simulink model "C172S_IntegratedAutopilot_V1"  (R2026a)
settings: Solver=ode4  StartTime=0  StopTime=180  FixedStep=0.01
InitFcn:
  | ah1Data = c172sLongitudinalData();
  | [~,ah1Plant] = c172sLongitudinalPlant(ah1Data);
  | ah1PitchController = c172sPitchAttitudeControllerData();
  | ah1Actuator = c172sElevatorActuatorData();
  | ah1AltitudeController = c172sAltitudeHoldControllerData();
  | A_ah1 = ah1Plant.A; B_ah1 = ah1Plant.B;
  | C_ah1 = ah1Plant.C; D_ah1 = ah1Plant.D;
  | Vtrim_ah1_mps = ah1Data.trim.V_mps;
  | Kh_ah1_per_s = ah1AltitudeController.altitudeGain_per_s;
  | Kv_ah1_radPerMps = ah1AltitudeController.verticalSpeedGain_radPerMps;
  | tauAltitude_ah1_s = ah1AltitudeController.commandFilterTimeConstant_s;
  | hDotLimit_ah1_mps = ah1AltitudeController.verticalSpeedCommandLimit_mps;
  | thetaLimit_ah1_rad = ah1AltitudeController.pitchCommandLimit_rad;
  | Kp_ah1 = ah1PitchController.Kp_radPerRad;
  | Ki_ah1_per_s = ah1PitchController.Ki_radPerRadPerS;
  | Kq_ah1_s = ah1Actuator.integration.Kq_s;
  | tauTheta_ah1_s = ah1PitchController.commandFilterTimeConstant_s;
  | tauActuator_ah1_s = ah1Actuator.dynamics.timeConstant_s;
  | Tt_ah1_s = ah1Actuator.antiWindup.trackingTimeConstant_s;
  | deltaELower_ah1_rad = ah1Actuator.authority.lowerLimit_rad;
  | deltaEUpper_ah1_rad = ah1Actuator.authority.upperLimit_rad;
  | deltaERate_ah1_radps = deg2rad(ah1Actuator.dynamics.rateLimit_degps);
  | if ~exist('hCommand_ah1_m','var'), hCommand_ah1_m = ah1AltitudeController.validation.operationalCommand_m; end
  | if ~exist('antiWindupEnable_ah1','var'), antiWindupEnable_ah1 = 1.0; end
  | if ~exist('x0_ah1','var'), x0_ah1 = zeros(4,1); end
  | if ~exist('xi0_ah1','var'), xi0_ah1 = 0.0; end
  | if ~exist('deltaE0_ah1','var'), deltaE0_ah1 = 0.0; end
  | if ~exist('h0_ah1_m','var'), h0_ah1_m = 0.0; end
  | hh1Data = c172sLateralDirectionalData();
  | [~,hh1Plant] = c172sLateralDirectionalPlant(hh1Data);
  | hh1YawController = c172sYawDamperData();
  | hh1RudderActuator = c172sRudderActuatorData();
  | hh1RollController = c172sRollAttitudeControllerData();
  | hh1AileronActuator = c172sAileronActuatorData();
  | hh1HeadingSensor = c172sHeadingSensorData();
  | hh1HeadingController = c172sHeadingHoldControllerData();
  | if ~strcmp(hh1Data.model.version,hh1HeadingController.requiredPlantVersion), error('HH V1 plant dependency mismatch.'); end
  | if ~strcmp(hh1YawController.artifactRevision,hh1HeadingController.requiredYawDamperRevision), error('HH V1 yaw-controller dependency mismatch.'); end
  | if ~strcmp(hh1RudderActuator.artifactRevision,hh1HeadingController.requiredRudderAuditRevision), error('HH V1 rudder-audit dependency mismatch.'); end
  | if ~strcmp(hh1AileronActuator.artifactRevision,hh1HeadingController.requiredAileronAuditRevision), error('HH V1 aileron-audit dependency mismatch.'); end
  | if ~strcmp(hh1RollController.artifactRevision,hh1HeadingController.requiredRollControllerRevision), error('HH V1 roll-controller dependency mismatch.'); end
  | if ~strcmp(hh1HeadingSensor.artifactRevision,hh1HeadingController.requiredHeadingSensorRevision), error('HH V1 heading-sensor dependency mismatch.'); end
  | A_hh1 = hh1Plant.A; B_hh1 = hh1Plant.B;
  | C_hh1 = hh1Plant.C; D_hh1 = hh1Plant.D;
  | Kphi_hh1 = hh1RollController.bankProportionalGain;
  | Ki_hh1 = hh1RollController.bankIntegralGain_per_s;
  | Kp_hh1 = hh1RollController.rollRateGain_s;
  | Tcmd_hh1 = hh1RollController.commandFilterTimeConstant_s;
  | Kr_hh1 = hh1YawController.rudderGain_s;
  | Tw_hh1 = hh1YawController.washoutTimeConstant_s;
  | TsRudder_hh1 = hh1RudderActuator.sensor.filterTimeConstant_s;
  | tauRudder_hh1 = hh1RudderActuator.dynamics.timeConstant_s;
  | TsRoll_hh1 = hh1AileronActuator.sensor.filterTimeConstant_s;
  | tauAileron_hh1 = hh1AileronActuator.dynamics.timeConstant_s;
  | Tt_hh1 = hh1AileronActuator.antiWindup.trackingTimeConstant_s;
  | delaySampleTime_hh1 = hh1AileronActuator.sensor.nominalDelay_s;
  | Kpsi_hh1 = hh1HeadingController.headingErrorGain;
  | TsHeading_hh1 = hh1HeadingSensor.filterTimeConstant_s;
  | headingDelaySampleTime_hh1 = hh1HeadingSensor.nominalDelay_s/5;
  | bankCommandLower_hh1_rad = -deg2rad(hh1HeadingController.bankCommandAuthority_deg);
  | bankCommandUpper_hh1_rad = deg2rad(hh1HeadingController.bankCommandAuthority_deg);
  | autoAileronLower_hh1_rad = hh1AileronActuator.authority.lowerLimit_rad;
  | autoAileronUpper_hh1_rad = hh1AileronActuator.authority.upperLimit_rad;
  | aileronRateLower_hh1_radps = -deg2rad(hh1AileronActuator.dynamics.rateLimit_degps);
  | aileronRateUpper_hh1_radps = deg2rad(hh1AileronActuator.dynamics.rateLimit_degps);
  | totalAileronLower_hh1_rad = hh1AileronActuator.physicalTravel.lowerLimit_rad;
  | totalAileronUpper_hh1_rad = hh1AileronActuator.physicalTravel.upperLimit_rad;
  | autoRudderLower_hh1_rad = hh1RudderActuator.authority.lowerLimit_rad;
  | autoRudderUpper_hh1_rad = hh1RudderActuator.authority.upperLimit_rad;
  | rudderRateLower_hh1_radps = -deg2rad(hh1RudderActuator.dynamics.rateLimit_degps);
  | rudderRateUpper_hh1_radps = deg2rad(hh1RudderActuator.dynamics.rateLimit_degps);
  | totalRudderLower_hh1_rad = hh1RudderActuator.physicalTravel.lowerLimit_rad;
  | totalRudderUpper_hh1_rad = hh1RudderActuator.physicalTravel.upperLimit_rad;
  | if ~exist('headingCommand_hh1_rad','var'), headingCommand_hh1_rad = deg2rad(30); end
  | if ~exist('headingBias_hh1_rad','var'), headingBias_hh1_rad = 0; end
  | if ~exist('headingNoiseAmplitude_hh1_rad','var'), headingNoiseAmplitude_hh1_rad = 0; end
  | if ~exist('headingNoiseFrequency_hh1_radps','var'), headingNoiseFrequency_hh1_radps = 0.8; end
  | if ~exist('pilotAileronBias_hh1_rad','var'), pilotAileronBias_hh1_rad = 0; end
  | if ~exist('pilotAileronPulse_hh1_rad','var'), pilotAileronPulse_hh1_rad = 0; end
  | if ~exist('pilotRudderBias_hh1_rad','var'), pilotRudderBias_hh1_rad = 0; end
  | if ~exist('pilotRudderPulse_hh1_rad','var'), pilotRudderPulse_hh1_rad = 0; end
  | if ~exist('aileronPulseStart_hh1_s','var'), aileronPulseStart_hh1_s = 5; end
  | if ~exist('aileronPulseEnd_hh1_s','var'), aileronPulseEnd_hh1_s = 6; end
  | if ~exist('rudderPulseStart_hh1_s','var'), rudderPulseStart_hh1_s = 5; end
  | if ~exist('rudderPulseEnd_hh1_s','var'), rudderPulseEnd_hh1_s = 6; end
  | if ~exist('pNoiseAmplitude_hh1_radps','var'), pNoiseAmplitude_hh1_radps = 0; end
  | if ~exist('pNoiseFrequency_hh1_radps','var'), pNoiseFrequency_hh1_radps = 50; end
  | if ~exist('phiNoiseAmplitude_hh1_rad','var'), phiNoiseAmplitude_hh1_rad = 0; end
  | if ~exist('phiNoiseFrequency_hh1_radps','var'), phiNoiseFrequency_hh1_radps = 5; end
  | if ~exist('yawNoiseAmplitude_hh1_radps','var'), yawNoiseAmplitude_hh1_radps = 0; end
  | if ~exist('yawNoiseFrequency_hh1_radps','var'), yawNoiseFrequency_hh1_radps = 50; end
  | if ~exist('antiWindupEnable_hh1','var'), antiWindupEnable_hh1 = 1; end
  | if ~exist('x0_hh1','var'), x0_hh1 = zeros(5,1); end
  | if ~exist('rDelay0_hh1_radps','var'), rDelay0_hh1_radps = x0_hh1(3); end
  | if ~exist('pDelay0_hh1_radps','var'), pDelay0_hh1_radps = x0_hh1(2); end
  | if ~exist('phiDelay0_hh1_rad','var'), phiDelay0_hh1_rad = x0_hh1(4); end
  | if ~exist('rSensor0_hh1_radps','var'), rSensor0_hh1_radps = 0; end
  | if ~exist('xw0_hh1_radps','var'), xw0_hh1_radps = 0; end
  | if ~exist('deltaRAuto0_hh1_rad','var'), deltaRAuto0_hh1_rad = 0; end
  | if ~exist('pSensor0_hh1_radps','var'), pSensor0_hh1_radps = 0; end
  | if ~exist('phiSensor0_hh1_rad','var'), phiSensor0_hh1_rad = 0; end
  | if ~exist('psiDelay0_hh1_rad','var'), psiDelay0_hh1_rad = x0_hh1(5); end
  | if ~exist('psiSensor0_hh1_rad','var'), psiSensor0_hh1_rad = x0_hh1(5)+headingBias_hh1_rad; end
  | if ~exist('xi0_hh1_rad_s','var'), xi0_hh1_rad_s = 0; end
  | if ~exist('deltaAAuto0_hh1_rad','var'), deltaAAuto0_hh1_rad = 0; end
  | if ~exist('filteredCommand0_hh1_rad','var'), filteredCommand0_hh1_rad = 0; end
  | ia1Integration = c172sIntegratedAutopilotData();
  | if ~strcmp(ia1Integration.artifactRevision,'INTEGRATED-AUTOPILOT-V1-INTERFACE-AUDIT-MATLAB-R1'), error('Integrated Autopilot V1 audit mismatch.'); end
  | if ~exist('ia1InputSignal','var'), error('ia1InputSignal is required.'); end
  | ia1TrimAltitude_ft = 4000.0;
undefined symbols (not defined in the file or in its folder): aileronPulseEnd_hh1_s, aileronPulseStart_hh1_s, antiWindupEnable_ah1, antiWindupEnable_hh1, deltaAAuto0_hh1_rad, deltaE0_ah1, deltaRAuto0_hh1_rad, filteredCommand0_hh1_rad, h0_ah1_m, headingBias_hh1_rad, headingNoiseAmplitude_hh1_rad, headingNoiseFrequency_hh1_radps, pDelay0_hh1_radps, phiDelay0_hh1_rad, phiNoiseAmplitude_hh1_rad, phiNoiseFrequency_hh1_radps, phiSensor0_hh1_rad, pilotAileronBias_hh1_rad, pilotAileronPulse_hh1_rad, pilotRudderBias_hh1_rad, pilotRudderPulse_hh1_rad, pNoiseAmplitude_hh1_radps, pNoiseFrequency_hh1_radps, pSensor0_hh1_radps, psiDelay0_hh1_rad, psiSensor0_hh1_rad, rDelay0_hh1_radps, rSensor0_hh1_radps, rudderPulseEnd_hh1_s, rudderPulseStart_hh1_s, x0_ah1, x0_hh1, xi0_ah1, xi0_hh1_rad_s, xw0_hh1_radps, yawNoiseAmplitude_hh1_radps, yawNoiseFrequency_hh1_radps
(part 1 of 2)
settings Model: Creator=Shahi  LastModifiedBy=Shahi

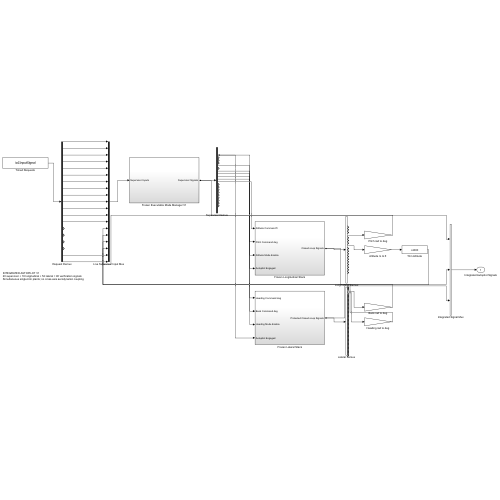
[thumbnail: Simulink's stored preview of the top-level diagram]
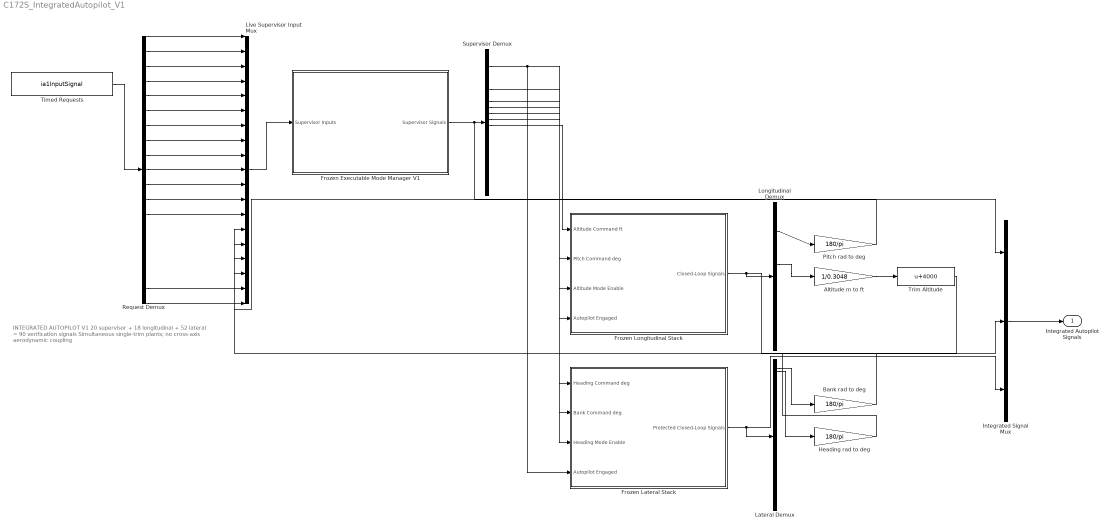
== system C172S_IntegratedAutopilot_V1 ==
  note: INTEGRATED AUTOPILOT V1
      | 20 supervisor + 18 longitudinal + 52 lateral = 90 verification signals
      | Simultaneous single-trim plants; no cross-axis aerodynamic coupling
  Altitude m to ft : Gain  Gain=1/0.3048
  Bank rad to deg : Gain  Gain=180/pi
  Frozen Executable Mode Manager V1 : Subsystem
  Frozen Lateral Stack : Subsystem
  Frozen Longitudinal Stack : Subsystem
  Heading rad to deg : Gain  Gain=180/pi
  Integrated Signal Mux : Mux  Inputs=3
  Lateral Demux : Demux  Outputs=52
  Live Supervisor Input Mux : Mux  Inputs=19
  Longitudinal Demux : Demux  Outputs=18
  Pitch rad to deg : Gain  Gain=180/pi
  Request Demux : Demux  Outputs=19
  Supervisor Demux : Demux  Outputs=20
  Timed Requests : FromWorkspace  VariableName=ia1InputSignal  SampleTime=0.01  Interpolate=off  OutputAfterFinalValue=Holding final value
  Trim Altitude : Bias  Bias=4000  SaturateOnIntegerOverflow=off
  Integrated Autopilot Signals : Outport
  wires:
  Timed Requests/1 -> Request Demux/1
  Frozen Longitudinal Stack/1(Closed-Loop Signals) -> Longitudinal Demux/1, Integrated Signal Mux/2
  Frozen Lateral Stack/1(Protected Closed-Loop Signals) -> Lateral Demux/1, Integrated Signal Mux/3
  Longitudinal Demux/4 -> Pitch rad to deg/1
  Longitudinal Demux/8 -> Altitude m to ft/1
  Altitude m to ft/1 -> Trim Altitude/1
  Lateral Demux/4 -> Bank rad to deg/1
  Lateral Demux/5 -> Heading rad to deg/1
  Request Demux/1 -> Live Supervisor Input Mux/1
  Request Demux/2 -> Live Supervisor Input Mux/2
  Request Demux/3 -> Live Supervisor Input Mux/3
  Request Demux/4 -> Live Supervisor Input Mux/4
  Request Demux/5 -> Live Supervisor Input Mux/5
  Request Demux/6 -> Live Supervisor Input Mux/6
  Request Demux/7 -> Live Supervisor Input Mux/7
  Request Demux/8 -> Live Supervisor Input Mux/8
  Request Demux/9 -> Live Supervisor Input Mux/9
  Request Demux/10 -> Live Supervisor Input Mux/10
  Request Demux/11 -> Live Supervisor Input Mux/11
  Request Demux/12 -> Live Supervisor Input Mux/12
  Request Demux/13 -> Live Supervisor Input Mux/13
  Request Demux/18 -> Live Supervisor Input Mux/18
  Request Demux/19 -> Live Supervisor Input Mux/19
  Bank rad to deg/1 -> Live Supervisor Input Mux/14
  Pitch rad to deg/1 -> Live Supervisor Input Mux/15
  Heading rad to deg/1 -> Live Supervisor Input Mux/16
  Trim Altitude/1 -> Live Supervisor Input Mux/17
  Live Supervisor Input Mux/1 -> Frozen Executable Mode Manager V1/1(Supervisor Inputs)
  Frozen Executable Mode Manager V1/1(Supervisor Signals) -> Supervisor Demux/1, Integrated Signal Mux/1
  Supervisor Demux/11 -> Frozen Longitudinal Stack/1(Altitude Command ft)
  Supervisor Demux/9 -> Frozen Longitudinal Stack/2(Pitch Command deg)
  Supervisor Demux/7 -> Frozen Longitudinal Stack/3(Altitude Mode Enable)
  Supervisor Demux/1 -> Frozen Longitudinal Stack/4(Autopilot Engaged), Frozen Lateral Stack/4(Autopilot Engaged)
  Supervisor Demux/10 -> Frozen Lateral Stack/1(Heading Command deg)
  Supervisor Demux/8 -> Frozen Lateral Stack/2(Bank Command deg)
  Supervisor Demux/5 -> Frozen Lateral Stack/3(Heading Mode Enable)
  Integrated Signal Mux/1 -> Integrated Autopilot Signals/1

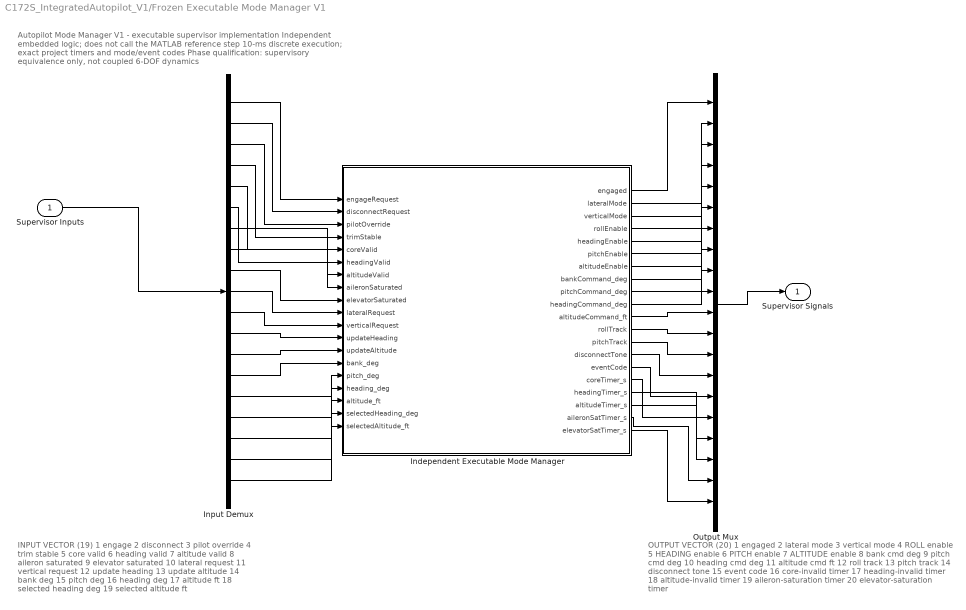
== system C172S_IntegratedAutopilot_V1/Frozen Executable Mode Manager V1 ==
  note: Autopilot Mode Manager V1 - executable supervisor implementation
      | Independent embedded logic; does not call the MATLAB reference step
      | 10-ms discrete execution; exact project timers and mode/event codes
      | Phase qualification: supervisory equivalence only, not coupled 6-DOF dynamics
  note: INPUT VECTOR (19)
      | 1 engage  2 disconnect  3 pilot override  4 trim stable
      | 5 core valid  6 heading valid  7 altitude valid
      | 8 aileron saturated  9 elevator saturated
      | 10 lateral request  11 vertical request
      | 12 update heading  13 update altitude
      | 14 bank deg  15 pitch deg  16 heading deg  17 altitude ft
      | 18 selected heading deg  19 selected altitude ft
  note: OUTPUT VECTOR (20)
      | 1 engaged  2 lateral mode  3 vertical mode
      | 4 ROLL enable  5 HEADING enable  6 PITCH enable  7 ALTITUDE enable
      | 8 bank cmd deg  9 pitch cmd deg  10 heading cmd deg  11 altitude cmd ft
      | 12 roll track  13 pitch track  14 disconnect tone  15 event code
      | 16 core-invalid timer  17 heading-invalid timer  18 altitude-invalid timer
      | 19 aileron-saturation timer  20 elevator-saturation timer
  Supervisor Inputs : Inport
  Independent Executable Mode Manager : MATLAB Function  TreatAsAtomicUnit=on
  Input Demux : Demux  Outputs=19
  Output Mux : Mux  Inputs=20
  Supervisor Signals : Outport
  wires:
  Input Demux/1 -> Independent Executable Mode Manager/1(engageRequest)
  Input Demux/2 -> Independent Executable Mode Manager/2(disconnectRequest)
  Input Demux/3 -> Independent Executable Mode Manager/3(pilotOverride)
  Input Demux/4 -> Independent Executable Mode Manager/4(trimStable)
  Input Demux/5 -> Independent Executable Mode Manager/5(coreValid)
  Input Demux/6 -> Independent Executable Mode Manager/6(headingValid)
  Input Demux/7 -> Independent Executable Mode Manager/7(altitudeValid)
  Input Demux/8 -> Independent Executable Mode Manager/8(aileronSaturated)
  Input Demux/9 -> Independent Executable Mode Manager/9(elevatorSaturated)
  Input Demux/10 -> Independent Executable Mode Manager/10(lateralRequest)
  Input Demux/11 -> Independent Executable Mode Manager/11(verticalRequest)
  Input Demux/12 -> Independent Executable Mode Manager/12(updateHeading)
  Input Demux/13 -> Independent Executable Mode Manager/13(updateAltitude)
  Input Demux/14 -> Independent Executable Mode Manager/14(bank_deg)
  Input Demux/15 -> Independent Executable Mode Manager/15(pitch_deg)
  Input Demux/16 -> Independent Executable Mode Manager/16(heading_deg)
  Input Demux/17 -> Independent Executable Mode Manager/17(altitude_ft)
  Input Demux/18 -> Independent Executable Mode Manager/18(selectedHeading_deg)
  Input Demux/19 -> Independent Executable Mode Manager/19(selectedAltitude_ft)
  Independent Executable Mode Manager/1(engaged) -> Output Mux/1
  Independent Executable Mode Manager/2(lateralMode) -> Output Mux/2
  Independent Executable Mode Manager/3(verticalMode) -> Output Mux/3
  Independent Executable Mode Manager/4(rollEnable) -> Output Mux/4
  Independent Executable Mode Manager/5(headingEnable) -> Output Mux/5
  Independent Executable Mode Manager/6(pitchEnable) -> Output Mux/6
  Independent Executable Mode Manager/7(altitudeEnable) -> Output Mux/7
  Independent Executable Mode Manager/8(bankCommand_deg) -> Output Mux/8
  Independent Executable Mode Manager/9(pitchCommand_deg) -> Output Mux/9
  Independent Executable Mode Manager/10(headingCommand_deg) -> Output Mux/10
  Independent Executable Mode Manager/11(altitudeCommand_ft) -> Output Mux/11
  Independent Executable Mode Manager/12(rollTrack) -> Output Mux/12
  Independent Executable Mode Manager/13(pitchTrack) -> Output Mux/13
  Independent Executable Mode Manager/14(disconnectTone) -> Output Mux/14
  Independent Executable Mode Manager/15(eventCode) -> Output Mux/15
  Independent Executable Mode Manager/16(coreTimer_s) -> Output Mux/16
  Independent Executable Mode Manager/17(headingTimer_s) -> Output Mux/17
  Independent Executable Mode Manager/18(altitudeTimer_s) -> Output Mux/18
  Independent Executable Mode Manager/19(aileronSatTimer_s) -> Output Mux/19
  Independent Executable Mode Manager/20(elevatorSatTimer_s) -> Output Mux/20
  Output Mux/1 -> Supervisor Signals/1
  Supervisor Inputs/1 -> Input Demux/1

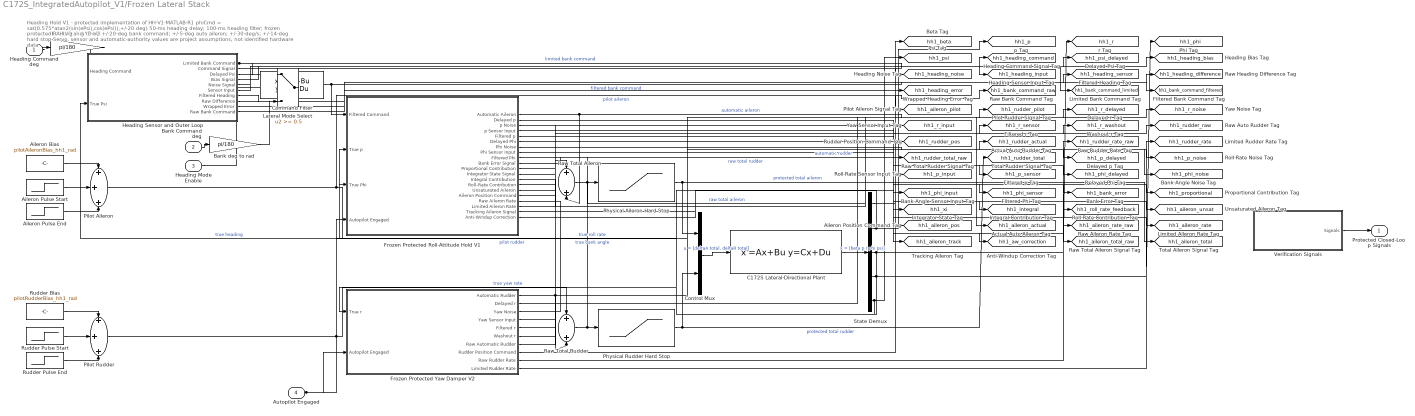
== system C172S_IntegratedAutopilot_V1/Frozen Lateral Stack ==
  note: Heading Hold V1 - protected implementation of HH-V1-MATLAB-R1
      | phiCmd = sat(0.575*atan2(sin(ePsi),cos(ePsi)),+/-20 deg)
      | 50-ms heading delay; 100-ms heading filter; frozen protected RAH V1 and YD V2
      | +/-20-deg bank command; +/-5-deg auto aileron; +/-30-deg/s; +/-14-deg hard stop
      | Servo, sensor and automatic-authority values are project assumptions, not identified hardware data
  Heading Command deg : Inport
  Bank Command deg : Inport  Port=2
  Heading Mode Enable : Inport  Port=3
  Autopilot Engaged : Inport  Port=4
  Aileron Bias : Constant  Value=pilotAileronBias_hh1_rad
  Aileron Pulse End : Step  Time=aileronPulseEnd_hh1_s  FinalValue=-pilotAileronPulse_hh1_rad  SampleTime=0
  Aileron Pulse Start : Step  Time=aileronPulseStart_hh1_s  FinalValue=pilotAileronPulse_hh1_rad  SampleTime=0
  Bank deg to rad : Gain  Gain=pi/180
  C172S Lateral-Directional Plant : StateSpace  A=A_hh1  B=B_hh1  C=C_hh1  D=D_hh1  InitialCondition=x0_hh1
  Command Filter : StateSpace  A=-1/Tcmd_hh1  B=1/Tcmd_hh1  D=0  InitialCondition=filteredCommand0_hh1_rad
  Control Mux : Mux  Inputs=2
  Frozen Protected Roll-Attitude Hold V1 : Subsystem
  Frozen Protected Yaw Damper V2 : Subsystem
  Heading Sensor and Outer Loop : Subsystem
  Heading deg to rad : Gain  Gain=pi/180
  Lateral Mode Select : Switch  Threshold=0.5  SaturateOnIntegerOverflow=off  InputSameDT=off
  Physical Aileron Hard Stop : Saturate  UpperLimit=totalAileronUpper_hh1_rad  LowerLimit=totalAileronLower_hh1_rad
  Physical Rudder Hard Stop : Saturate  UpperLimit=totalRudderUpper_hh1_rad  LowerLimit=totalRudderLower_hh1_rad
  Pilot Aileron : Sum  Inputs=+++
  Pilot Rudder : Sum  Inputs=+++
  Raw Total Aileron : Sum
  Raw Total Rudder : Sum
  Rudder Bias : Constant  Value=pilotRudderBias_hh1_rad
  Rudder Pulse End : Step  Time=rudderPulseEnd_hh1_s  FinalValue=-pilotRudderPulse_hh1_rad  SampleTime=0
  Rudder Pulse Start : Step  Time=rudderPulseStart_hh1_s  FinalValue=pilotRudderPulse_hh1_rad  SampleTime=0
  State Demux : Demux  Outputs=5
  Verification Signals : Subsystem
  Protected Closed-Loop Signals : Outport
  tag scope: hh1_aileron_actual=global, hh1_aileron_pilot=global, hh1_aileron_pos=global, hh1_aileron_rate=global, hh1_aileron_rate_raw=global, hh1_aileron_total=global, hh1_aileron_total_raw=global, hh1_aileron_track=global, hh1_aileron_unsat=global, hh1_aw_correction=global, hh1_bank_command_filtered=global, hh1_bank_command_limited=global, hh1_bank_command_raw=global, hh1_bank_error=global, hh1_beta=global, hh1_heading_bias=global, hh1_heading_command=global, hh1_heading_difference=global, hh1_heading_error=global, hh1_heading_input=global, hh1_heading_noise=global, hh1_heading_sensor=global, hh1_integral=global, hh1_p=global, hh1_p_delayed=global, hh1_p_input=global, hh1_p_noise=global, hh1_p_sensor=global, hh1_phi=global, hh1_phi_delayed=global, hh1_phi_input=global, hh1_phi_noise=global, hh1_phi_sensor=global, hh1_proportional=global, hh1_psi=global, hh1_psi_delayed=global, hh1_r=global, hh1_r_delayed=global, hh1_r_input=global, hh1_r_noise=global, hh1_r_sensor=global, hh1_r_washout=global, hh1_roll_rate_feedback=global, hh1_rudder_actual=global, hh1_rudder_pilot=global, hh1_rudder_pos=global, hh1_rudder_rate=global, hh1_rudder_rate_raw=global, hh1_rudder_raw=global, hh1_rudder_total=global, hh1_rudder_total_raw=global, hh1_xi=global
  wires:
  Heading Sensor and Outer Loop/1(Limited Bank Command) -> [hh1_bank_command_limited], Lateral Mode Select/1  "limited bank command"
  Command Filter/1 -> [hh1_bank_command_filtered], Frozen Protected Roll-Attitude Hold V1/1(Filtered Command)  "filtered bank command"
  Aileron Bias/1 -> Pilot Aileron/1
  Aileron Pulse Start/1 -> Pilot Aileron/2
  Aileron Pulse End/1 -> Pilot Aileron/3
  Rudder Bias/1 -> Pilot Rudder/1
  Rudder Pulse Start/1 -> Pilot Rudder/2
  Rudder Pulse End/1 -> Pilot Rudder/3
  Pilot Aileron/1 -> [hh1_aileron_pilot], Raw Total Aileron/1  "pilot aileron"
  Frozen Protected Roll-Attitude Hold V1/1(Automatic Aileron) -> [hh1_aileron_actual], Raw Total Aileron/2  "automatic aileron"
  Raw Total Aileron/1 -> [hh1_aileron_total_raw], Physical Aileron Hard Stop/1  "raw total aileron"
  Physical Aileron Hard Stop/1 -> [hh1_aileron_total], Control Mux/1  "protected total aileron"
  Pilot Rudder/1 -> [hh1_rudder_pilot], Raw Total Rudder/1  "pilot rudder"
  Frozen Protected Yaw Damper V2/1(Automatic Rudder) -> [hh1_rudder_actual], Raw Total Rudder/2  "automatic rudder"
  Raw Total Rudder/1 -> [hh1_rudder_total_raw], Physical Rudder Hard Stop/1  "raw total rudder"
  Physical Rudder Hard Stop/1 -> [hh1_rudder_total], Control Mux/2  "protected total rudder"
  Control Mux/1 -> C172S Lateral-Directional Plant/1  "u = [deltaA total, deltaR total]"
  C172S Lateral-Directional Plant/1 -> State Demux/1  "x = [beta p r phi psi]"
  State Demux/2 -> [hh1_p], Frozen Protected Roll-Attitude Hold V1/2(True p)  "true roll rate"
  State Demux/4 -> [hh1_phi], Frozen Protected Roll-Attitude Hold V1/3(True Phi)  "true bank angle"
  State Demux/3 -> [hh1_r], Frozen Protected Yaw Damper V2/1(True r)  "true yaw rate"
  State Demux/5 -> [hh1_psi], Heading Sensor and Outer Loop/2(True Psi)  "true heading"
  Verification Signals/1(Signals) -> Protected Closed-Loop Signals/1
  State Demux/1 -> [hh1_beta]
  Heading Sensor and Outer Loop/2(Command Signal) -> [hh1_heading_command]
  Heading Sensor and Outer Loop/3(Delayed Psi) -> [hh1_psi_delayed]
  Heading Sensor and Outer Loop/4(Bias Signal) -> [hh1_heading_bias]
  Heading Sensor and Outer Loop/5(Noise Signal) -> [hh1_heading_noise]
  Heading Sensor and Outer Loop/6(Sensor Input) -> [hh1_heading_input]
  Heading Sensor and Outer Loop/7(Filtered Heading) -> [hh1_heading_sensor]
  Heading Sensor and Outer Loop/8(Raw Difference) -> [hh1_heading_difference]
  Heading Sensor and Outer Loop/9(Wrapped Error) -> [hh1_heading_error]
  Heading Sensor and Outer Loop/10(Raw Bank Command) -> [hh1_bank_command_raw]
  Frozen Protected Yaw Damper V2/2(Delayed r) -> [hh1_r_delayed]
  Frozen Protected Yaw Damper V2/3(Yaw Noise) -> [hh1_r_noise]
  Frozen Protected Yaw Damper V2/4(Yaw Sensor Input) -> [hh1_r_input]
  Frozen Protected Yaw Damper V2/5(Filtered r) -> [hh1_r_sensor]
  Frozen Protected Yaw Damper V2/6(Washout r) -> [hh1_r_washout]
  Frozen Protected Yaw Damper V2/7(Raw Automatic Rudder) -> [hh1_rudder_raw]
  Frozen Protected Yaw Damper V2/8(Rudder Position Command) -> [hh1_rudder_pos]
  Frozen Protected Yaw Damper V2/9(Raw Rudder Rate) -> [hh1_rudder_rate_raw]
  Frozen Protected Yaw Damper V2/10(Limited Rudder Rate) -> [hh1_rudder_rate]
  Frozen Protected Roll-Attitude Hold V1/2(Delayed p) -> [hh1_p_delayed]
  Frozen Protected Roll-Attitude Hold V1/3(p Noise) -> [hh1_p_noise]
  Frozen Protected Roll-Attitude Hold V1/4(p Sensor Input) -> [hh1_p_input]
  Frozen Protected Roll-Attitude Hold V1/5(Filtered p) -> [hh1_p_sensor]
  Frozen Protected Roll-Attitude Hold V1/6(Delayed Phi) -> [hh1_phi_delayed]
  Frozen Protected Roll-Attitude Hold V1/7(Phi Noise) -> [hh1_phi_noise]
  Frozen Protected Roll-Attitude Hold V1/8(Phi Sensor Input) -> [hh1_phi_input]
  Frozen Protected Roll-Attitude Hold V1/9(Filtered Phi) -> [hh1_phi_sensor]
  Frozen Protected Roll-Attitude Hold V1/10(Bank Error Signal) -> [hh1_bank_error]
  Frozen Protected Roll-Attitude Hold V1/11(Proportional Contribution) -> [hh1_proportional]
  Frozen Protected Roll-Attitude Hold V1/12(Integrator State Signal) -> [hh1_xi]
  Frozen Protected Roll-Attitude Hold V1/13(Integral Contribution) -> [hh1_integral]
  Frozen Protected Roll-Attitude Hold V1/14(Roll-Rate Contribution) -> [hh1_roll_rate_feedback]
  Frozen Protected Roll-Attitude Hold V1/15(Unsaturated Aileron) -> [hh1_aileron_unsat]
  Frozen Protected Roll-Attitude Hold V1/16(Aileron Position Command) -> [hh1_aileron_pos]
  Frozen Protected Roll-Attitude Hold V1/17(Raw Aileron Rate) -> [hh1_aileron_rate_raw]
  Frozen Protected Roll-Attitude Hold V1/18(Limited Aileron Rate) -> [hh1_aileron_rate]
  Frozen Protected Roll-Attitude Hold V1/19(Tracking Aileron Signal) -> [hh1_aileron_track]
  Frozen Protected Roll-Attitude Hold V1/20(Anti-Windup Correction) -> [hh1_aw_correction]
  Heading Command deg/1 -> Heading deg to rad/1
  Heading deg to rad/1 -> Heading Sensor and Outer Loop/1(Heading Command)
  Bank Command deg/1 -> Bank deg to rad/1
  Heading Mode Enable/1 -> Lateral Mode Select/2
  Bank deg to rad/1 -> Lateral Mode Select/3
  Lateral Mode Select/1 -> Command Filter/1
  Autopilot Engaged/1 -> Frozen Protected Roll-Attitude Hold V1/4(Autopilot Engaged), Frozen Protected Yaw Damper V2/2(Autopilot Engaged)

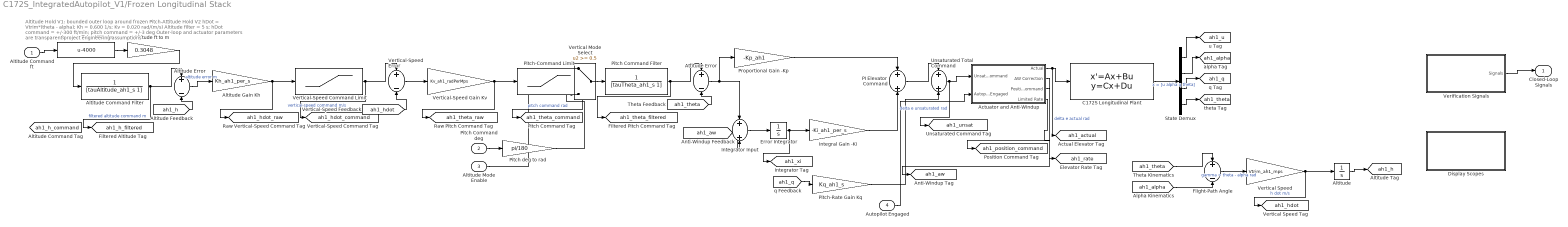
== system C172S_IntegratedAutopilot_V1/Frozen Longitudinal Stack ==
  note: Altitude Hold V1: bounded outer loop around frozen Pitch-Attitude Hold V2
      | hDot = Vtrim*(theta - alpha); Kh = 0.600 1/s; Kv = 0.020 rad/(m/s)
      | Altitude filter = 5 s; hDot command = +/-300 ft/min; pitch command = +/-3 deg
      | Outer-loop and actuator parameters are transparent project engineering assumptions
  Altitude Command ft : Inport
  Pitch Command deg : Inport  Port=2
  Altitude Mode Enable : Inport  Port=3
  Autopilot Engaged : Inport  Port=4
  Actuator and Anti-Windup : Subsystem
  Altitude : Integrator  InitialCondition=h0_ah1_m
  Altitude Command Filter : TransferFcn  Numerator=1  Denominator=[tauAltitude_ah1_s 1]
  Altitude Error : Sum  Inputs=+-
  Altitude Gain Kh : Gain  Gain=Kh_ah1_per_s
  Altitude ft to m : Gain  Gain=0.3048
  Attitude Error : Sum  Inputs=+-
  C172S Longitudinal Plant : StateSpace  A=A_ah1  B=B_ah1  C=C_ah1  D=D_ah1  InitialCondition=x0_ah1
  Display Scopes : Subsystem
  Error Integrator : Integrator  InitialCondition=xi0_ah1
  Flight-Path Angle : Sum  Inputs=+-
  Integral Gain -Ki : Gain  Gain=-Ki_ah1_per_s
  Integrator Input : Sum
  PI Elevator Command : Sum
  Pitch Command Filter : TransferFcn  Numerator=1  Denominator=[tauTheta_ah1_s 1]
  Pitch deg to rad : Gain  Gain=pi/180
  Pitch-Command Limit : Saturate  UpperLimit=thetaLimit_ah1_rad  LowerLimit=-thetaLimit_ah1_rad
  Pitch-Rate Gain Kq : Gain  Gain=Kq_ah1_s
  Proportional Gain -Kp : Gain  Gain=-Kp_ah1
  Remove Trim Altitude : Bias  Bias=-4000  SaturateOnIntegerOverflow=off
  State Demux : Demux
  Unsaturated Total Command : Sum
  Verification Signals : Subsystem
  Vertical Mode Select : Switch  Threshold=0.5  SaturateOnIntegerOverflow=off  InputSameDT=off
  Vertical Speed : Gain  Gain=Vtrim_ah1_mps
  Vertical-Speed Command Limit : Saturate  UpperLimit=hDotLimit_ah1_mps  LowerLimit=-hDotLimit_ah1_mps
  Vertical-Speed Error : Sum  Inputs=+-
  Vertical-Speed Gain Kv : Gain  Gain=Kv_ah1_radPerMps
  Closed-Loop Signals : Outport
  tag scope: ah1_actual=global, ah1_alpha=global, ah1_aw=global, ah1_h=global, ah1_h_command=global, ah1_h_filtered=global, ah1_hdot=global, ah1_hdot_command=global, ah1_hdot_raw=global, ah1_position_command=global, ah1_q=global, ah1_rate=global, ah1_theta=global, ah1_theta_command=global, ah1_theta_filtered=global, ah1_theta_raw=global, ah1_u=global, ah1_unsat=global, ah1_xi=global
  wires:
  ? -> [ah1_h_command]  "altitude command m"
  Altitude Command Filter/1 -> [ah1_h_filtered], Altitude Error/1  "filtered altitude command m"
  [ah1_h] -> Altitude Error/2
  Altitude Error/1 -> Altitude Gain Kh/1  "altitude error m"
  Altitude Gain Kh/1 -> [ah1_hdot_raw], Vertical-Speed Command Limit/1
  Vertical-Speed Command Limit/1 -> [ah1_hdot_command], Vertical-Speed Error/1  "vertical-speed command m/s"
  [ah1_hdot] -> Vertical-Speed Error/2
  Vertical-Speed Error/1 -> Vertical-Speed Gain Kv/1
  Vertical-Speed Gain Kv/1 -> [ah1_theta_raw], Pitch-Command Limit/1
  Pitch-Command Limit/1 -> [ah1_theta_command], Vertical Mode Select/1  "pitch command rad"
  Pitch Command Filter/1 -> [ah1_theta_filtered], Attitude Error/1
  [ah1_theta] -> Attitude Error/2
  Attitude Error/1 -> Integrator Input/1, Proportional Gain -Kp/1
  [ah1_aw] -> Integrator Input/2
  Integrator Input/1 -> Error Integrator/1
  Error Integrator/1 -> [ah1_xi], Integral Gain -Ki/1
  Proportional Gain -Kp/1 -> PI Elevator Command/1
  Integral Gain -Ki/1 -> PI Elevator Command/2
  [ah1_q] -> Pitch-Rate Gain Kq/1
  PI Elevator Command/1 -> Unsaturated Total Command/1
  Pitch-Rate Gain Kq/1 -> Unsaturated Total Command/2
  Unsaturated Total Command/1 -> [ah1_unsat], Actuator and Anti-Windup/1(Unsaturated Command)  "delta e unsaturated rad"
  Actuator and Anti-Windup/1(Actual) -> [ah1_actual], C172S Longitudinal Plant/1  "delta e actual rad"
  C172S Longitudinal Plant/1 -> State Demux/1  "x = [u alpha q theta]"
  [ah1_theta] -> Flight-Path Angle/1
  [ah1_alpha] -> Flight-Path Angle/2
  Flight-Path Angle/1 -> Vertical Speed/1  "gamma = theta - alpha rad"
  Vertical Speed/1 -> [ah1_hdot], Altitude/1  "h dot m/s"
  Actuator and Anti-Windup/2(AW Correction) -> [ah1_aw]
  Actuator and Anti-Windup/3(Position Command) -> [ah1_position_command]
  Actuator and Anti-Windup/4(Limited Rate) -> [ah1_rate]
  Altitude/1 -> [ah1_h]
  State Demux/1 -> [ah1_u]
  State Demux/2 -> [ah1_alpha]
  State Demux/3 -> [ah1_q]
  State Demux/4 -> [ah1_theta]
  Verification Signals/1(Signals) -> Closed-Loop Signals/1
  Altitude Command ft/1 -> Remove Trim Altitude/1
  Remove Trim Altitude/1 -> Altitude ft to m/1
  Altitude ft to m/1 -> Altitude Command Filter/1
  Pitch Command deg/1 -> Pitch deg to rad/1
  Altitude Mode Enable/1 -> Vertical Mode Select/2
  Pitch deg to rad/1 -> Vertical Mode Select/3
  Vertical Mode Select/1 -> Pitch Command Filter/1
  Autopilot Engaged/1 -> Actuator and Anti-Windup/2(Autopilot Engaged)

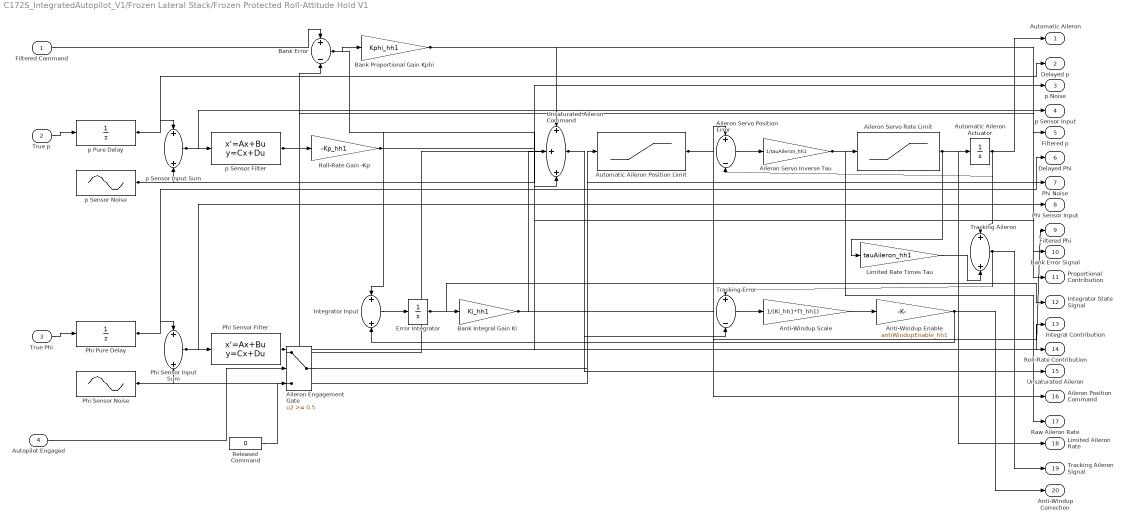
== system C172S_IntegratedAutopilot_V1/Frozen Lateral Stack/Frozen Protected Roll-Attitude Hold V1 ==
  Filtered Command : Inport
  True p : Inport  Port=2
  True Phi : Inport  Port=3
  Autopilot Engaged : Inport  Port=4
  Aileron Engagement Gate : Switch  Threshold=0.5  SaturateOnIntegerOverflow=off  InputSameDT=off
  Aileron Servo Inverse Tau : Gain  Gain=1/tauAileron_hh1
  Aileron Servo Position Error : Sum  Inputs=+-
  Aileron Servo Rate Limit : Saturate  UpperLimit=aileronRateUpper_hh1_radps  LowerLimit=aileronRateLower_hh1_radps
  Anti-Windup Enable : Gain  Gain=antiWindupEnable_hh1
  Anti-Windup Scale : Gain  Gain=1/(Ki_hh1*Tt_hh1)
  Automatic Aileron Actuator : Integrator  InitialCondition=deltaAAuto0_hh1_rad
  Automatic Aileron Position Limit : Saturate  UpperLimit=autoAileronUpper_hh1_rad  LowerLimit=autoAileronLower_hh1_rad
  Bank Error : Sum  Inputs=+-
  Bank Integral Gain Ki : Gain  Gain=Ki_hh1
  Bank Proportional Gain Kphi : Gain  Gain=Kphi_hh1
  Error Integrator : Integrator  InitialCondition=xi0_hh1_rad_s
  Integrator Input : Sum
  Limited Rate Times Tau : Gain  Gain=tauAileron_hh1
  Phi Pure Delay : UnitDelay  InitialCondition=phiDelay0_hh1_rad  SampleTime=delaySampleTime_hh1
  Phi Sensor Filter : StateSpace  A=-1/TsRoll_hh1  B=1/TsRoll_hh1  D=0  InitialCondition=phiSensor0_hh1_rad
  Phi Sensor Input Sum : Sum
  Phi Sensor Noise : Sin  Amplitude=phiNoiseAmplitude_hh1_rad  Frequency=phiNoiseFrequency_hh1_radps  SampleTime=0
  Released Command : Constant  Value=0
  Roll-Rate Gain -Kp : Gain  Gain=-Kp_hh1
  Tracking Aileron : Sum
  Tracking Error : Sum  Inputs=+-
  Unsaturated Aileron Command : Sum  Inputs=+++
  p Pure Delay : UnitDelay  InitialCondition=pDelay0_hh1_radps  SampleTime=delaySampleTime_hh1
  p Sensor Filter : StateSpace  A=-1/TsRoll_hh1  B=1/TsRoll_hh1  D=0  InitialCondition=pSensor0_hh1_radps
  p Sensor Input Sum : Sum
  p Sensor Noise : Sin  Amplitude=pNoiseAmplitude_hh1_radps  Frequency=pNoiseFrequency_hh1_radps  SampleTime=0
  Automatic Aileron : Outport
  Delayed p : Outport  Port=2
  p Noise : Outport  Port=3
  p Sensor Input : Outport  Port=4
  Filtered p : Outport  Port=5
  Delayed Phi : Outport  Port=6
  Phi Noise : Outport  Port=7
  Phi Sensor Input : Outport  Port=8
  Filtered Phi : Outport  Port=9
  Bank Error Signal : Outport  Port=10
  Proportional Contribution : Outport  Port=11
  Integrator State Signal : Outport  Port=12
  Integral Contribution : Outport  Port=13
  Roll-Rate Contribution : Outport  Port=14
  Unsaturated Aileron : Outport  Port=15
  Aileron Position Command : Outport  Port=16
  Raw Aileron Rate : Outport  Port=17
  Limited Aileron Rate : Outport  Port=18
  Tracking Aileron Signal : Outport  Port=19
  Anti-Windup Correction : Outport  Port=20
  wires:
  Anti-Windup Enable/1 -> Anti-Windup Correction/1, Integrator Input/2
  Anti-Windup Scale/1 -> Anti-Windup Enable/1
  Tracking Error/1 -> Anti-Windup Scale/1
  Tracking Aileron/1 -> Tracking Aileron Signal/1, Tracking Error/1
  Limited Rate Times Tau/1 -> Tracking Aileron/2
  Aileron Servo Rate Limit/1 -> Limited Aileron Rate/1, Limited Rate Times Tau/1, Automatic Aileron Actuator/1
  Aileron Servo Inverse Tau/1 -> Raw Aileron Rate/1, Aileron Servo Rate Limit/1
  Aileron Servo Position Error/1 -> Aileron Servo Inverse Tau/1
  Automatic Aileron Actuator/1 -> Automatic Aileron/1, Tracking Aileron/1, Aileron Servo Position Error/2
  Automatic Aileron Position Limit/1 -> Aileron Position Command/1, Aileron Servo Position Error/1
  Unsaturated Aileron Command/1 -> Unsaturated Aileron/1, Tracking Error/2, Aileron Engagement Gate/1
  Roll-Rate Gain -Kp/1 -> Roll-Rate Contribution/1, Unsaturated Aileron Command/3
  Bank Integral Gain Ki/1 -> Integral Contribution/1, Unsaturated Aileron Command/2
  Bank Proportional Gain Kphi/1 -> Proportional Contribution/1, Unsaturated Aileron Command/1
  Error Integrator/1 -> Integrator State Signal/1, Bank Integral Gain Ki/1
  Integrator Input/1 -> Error Integrator/1
  Bank Error/1 -> Bank Error Signal/1, Integrator Input/1, Bank Proportional Gain Kphi/1
  Phi Sensor Filter/1 -> Filtered Phi/1, Bank Error/2
  Filtered Command/1 -> Bank Error/1
  Phi Sensor Input Sum/1 -> Phi Sensor Input/1, Phi Sensor Filter/1
  Phi Sensor Noise/1 -> Phi Noise/1, Phi Sensor Input Sum/2
  Phi Pure Delay/1 -> Delayed Phi/1, Phi Sensor Input Sum/1
  True Phi/1 -> Phi Pure Delay/1
  p Sensor Filter/1 -> Filtered p/1, Roll-Rate Gain -Kp/1
  p Sensor Input Sum/1 -> p Sensor Input/1, p Sensor Filter/1
  p Sensor Noise/1 -> p Noise/1, p Sensor Input Sum/2
  p Pure Delay/1 -> Delayed p/1, p Sensor Input Sum/1
  True p/1 -> p Pure Delay/1
  Autopilot Engaged/1 -> Aileron Engagement Gate/2
  Released Command/1 -> Aileron Engagement Gate/3
  Aileron Engagement Gate/1 -> Automatic Aileron Position Limit/1

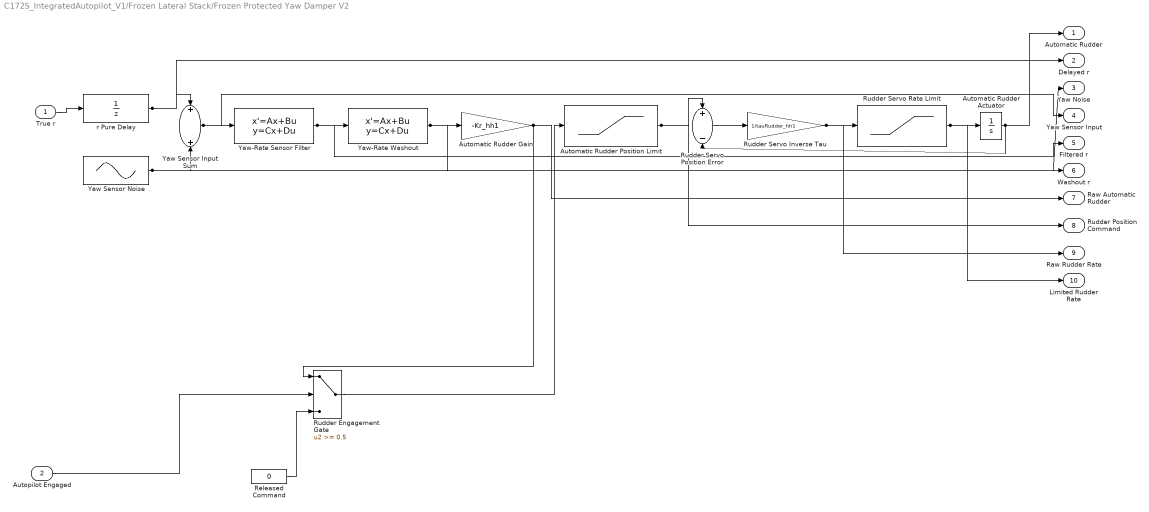
== system C172S_IntegratedAutopilot_V1/Frozen Lateral Stack/Frozen Protected Yaw Damper V2 ==
  True r : Inport
  Autopilot Engaged : Inport  Port=2
  Automatic Rudder Actuator : Integrator  InitialCondition=deltaRAuto0_hh1_rad
  Automatic Rudder Gain : Gain  Gain=-Kr_hh1
  Automatic Rudder Position Limit : Saturate  UpperLimit=autoRudderUpper_hh1_rad  LowerLimit=autoRudderLower_hh1_rad
  Released Command : Constant  Value=0
  Rudder Engagement Gate : Switch  Threshold=0.5  SaturateOnIntegerOverflow=off  InputSameDT=off
  Rudder Servo Inverse Tau : Gain  Gain=1/tauRudder_hh1
  Rudder Servo Position Error : Sum  Inputs=+-
  Rudder Servo Rate Limit : Saturate  UpperLimit=rudderRateUpper_hh1_radps  LowerLimit=rudderRateLower_hh1_radps
  Yaw Sensor Input Sum : Sum
  Yaw Sensor Noise : Sin  Amplitude=yawNoiseAmplitude_hh1_radps  Frequency=yawNoiseFrequency_hh1_radps  SampleTime=0
  Yaw-Rate Sensor Filter : StateSpace  A=-1/TsRudder_hh1  B=1/TsRudder_hh1  D=0  InitialCondition=rSensor0_hh1_radps
  Yaw-Rate Washout : StateSpace  A=-1/Tw_hh1  B=1/Tw_hh1  C=-1  InitialCondition=xw0_hh1_radps
  r Pure Delay : UnitDelay  InitialCondition=rDelay0_hh1_radps  SampleTime=delaySampleTime_hh1
  Automatic Rudder : Outport
  Delayed r : Outport  Port=2
  Yaw Noise : Outport  Port=3
  Yaw Sensor Input : Outport  Port=4
  Filtered r : Outport  Port=5
  Washout r : Outport  Port=6
  Raw Automatic Rudder : Outport  Port=7
  Rudder Position Command : Outport  Port=8
  Raw Rudder Rate : Outport  Port=9
  Limited Rudder Rate : Outport  Port=10
  wires:
  Rudder Servo Rate Limit/1 -> Limited Rudder Rate/1, Automatic Rudder Actuator/1
  Rudder Servo Inverse Tau/1 -> Raw Rudder Rate/1, Rudder Servo Rate Limit/1
  Rudder Servo Position Error/1 -> Rudder Servo Inverse Tau/1
  Automatic Rudder Actuator/1 -> Automatic Rudder/1, Rudder Servo Position Error/2
  Automatic Rudder Position Limit/1 -> Rudder Position Command/1, Rudder Servo Position Error/1
  Automatic Rudder Gain/1 -> Raw Automatic Rudder/1, Rudder Engagement Gate/1
  Yaw-Rate Washout/1 -> Washout r/1, Automatic Rudder Gain/1
  Yaw-Rate Sensor Filter/1 -> Filtered r/1, Yaw-Rate Washout/1
  Yaw Sensor Input Sum/1 -> Yaw Sensor Input/1, Yaw-Rate Sensor Filter/1
  Yaw Sensor Noise/1 -> Yaw Noise/1, Yaw Sensor Input Sum/2
  r Pure Delay/1 -> Delayed r/1, Yaw Sensor Input Sum/1
  True r/1 -> r Pure Delay/1
  Autopilot Engaged/1 -> Rudder Engagement Gate/2
  Released Command/1 -> Rudder Engagement Gate/3
  Rudder Engagement Gate/1 -> Automatic Rudder Position Limit/1

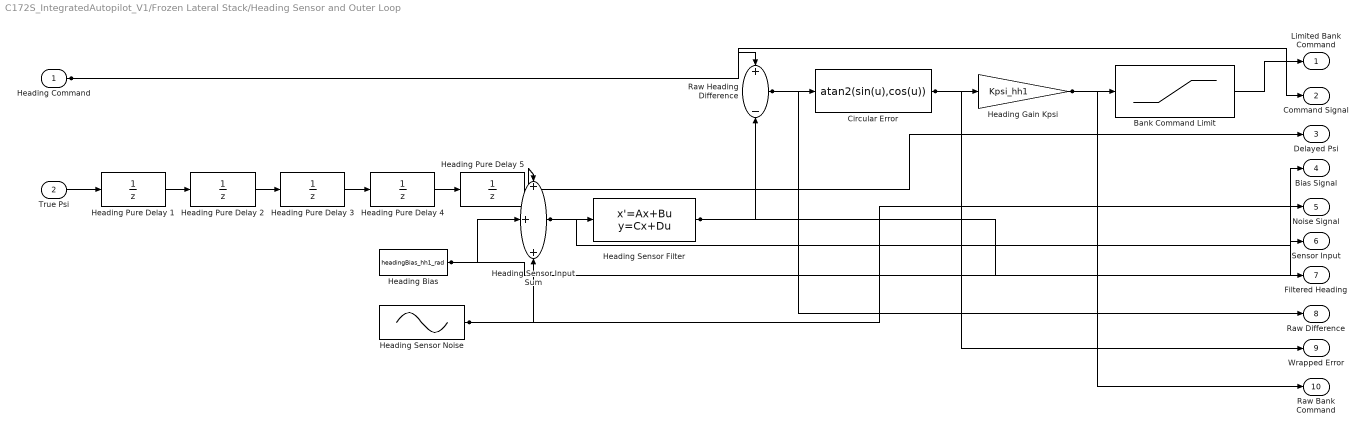
== system C172S_IntegratedAutopilot_V1/Frozen Lateral Stack/Heading Sensor and Outer Loop ==
  Heading Command : Inport
  True Psi : Inport  Port=2
  Bank Command Limit : Saturate  UpperLimit=bankCommandUpper_hh1_rad  LowerLimit=bankCommandLower_hh1_rad
  Circular Error : Fcn  Expr=atan2(sin(u),cos(u))
  Heading Bias : Constant  Value=headingBias_hh1_rad
  Heading Gain Kpsi : Gain  Gain=Kpsi_hh1
  Heading Pure Delay {1..5} (5 alike) : UnitDelay  InitialCondition=psiDelay0_hh1_rad  SampleTime=headingDelaySampleTime_hh1
  Heading Sensor Filter : StateSpace  A=-1/TsHeading_hh1  B=1/TsHeading_hh1  D=0  InitialCondition=psiSensor0_hh1_rad
  Heading Sensor Input Sum : Sum  Inputs=+++
  Heading Sensor Noise : Sin  Amplitude=headingNoiseAmplitude_hh1_rad  Frequency=headingNoiseFrequency_hh1_radps  SampleTime=0
  Raw Heading Difference : Sum  Inputs=+-
  Limited Bank Command : Outport
  Command Signal : Outport  Port=2
  Delayed Psi : Outport  Port=3
  Bias Signal : Outport  Port=4
  Noise Signal : Outport  Port=5
  Sensor Input : Outport  Port=6
  Filtered Heading : Outport  Port=7
  Raw Difference : Outport  Port=8
  Wrapped Error : Outport  Port=9
  Raw Bank Command : Outport  Port=10
  wires:
  Bank Command Limit/1 -> Limited Bank Command/1
  Heading Gain Kpsi/1 -> Raw Bank Command/1, Bank Command Limit/1
  Circular Error/1 -> Wrapped Error/1, Heading Gain Kpsi/1
  Raw Heading Difference/1 -> Raw Difference/1, Circular Error/1
  Heading Sensor Filter/1 -> Filtered Heading/1, Raw Heading Difference/2
  Heading Command/1 -> Command Signal/1, Raw Heading Difference/1
  Heading Sensor Input Sum/1 -> Sensor Input/1, Heading Sensor Filter/1
  Heading Sensor Noise/1 -> Noise Signal/1, Heading Sensor Input Sum/3
  Heading Bias/1 -> Bias Signal/1, Heading Sensor Input Sum/2
  Heading Pure Delay 5/1 -> Delayed Psi/1, Heading Sensor Input Sum/1
  Heading Pure Delay 4/1 -> Heading Pure Delay 5/1
  Heading Pure Delay 3/1 -> Heading Pure Delay 4/1
  Heading Pure Delay 2/1 -> Heading Pure Delay 3/1
  Heading Pure Delay 1/1 -> Heading Pure Delay 2/1
  True Psi/1 -> Heading Pure Delay 1/1

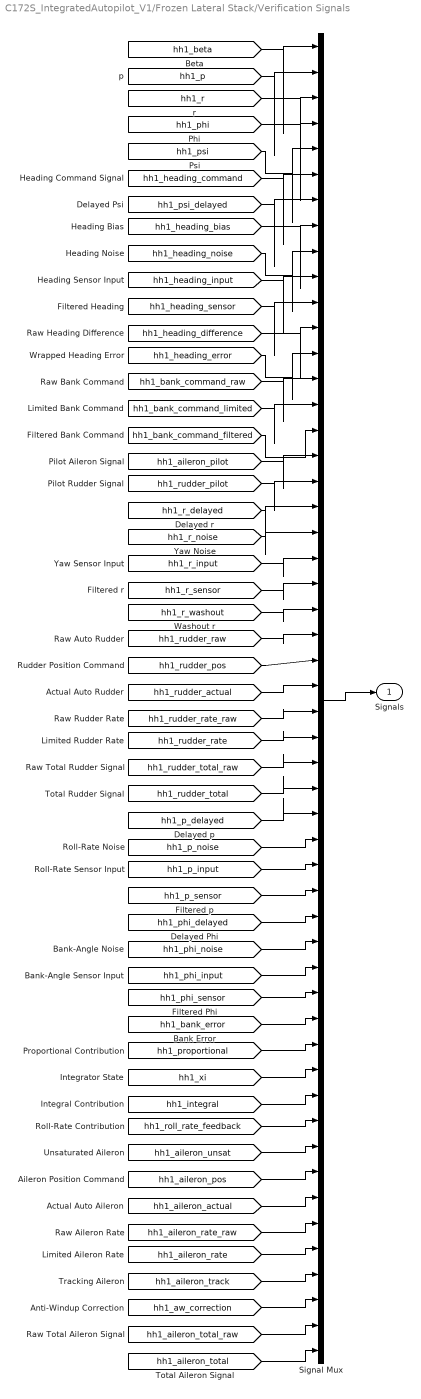
== system C172S_IntegratedAutopilot_V1/Frozen Lateral Stack/Verification Signals ==
  Signal Mux : Mux  Inputs=52
  Signals : Outport
  wires:
  Signal Mux/1 -> Signals/1
  [hh1_aileron_total] -> Signal Mux/52
  [hh1_aileron_total_raw] -> Signal Mux/51
  [hh1_aw_correction] -> Signal Mux/50
  [hh1_aileron_track] -> Signal Mux/49
  [hh1_aileron_rate] -> Signal Mux/48
  [hh1_aileron_rate_raw] -> Signal Mux/47
  [hh1_aileron_actual] -> Signal Mux/46
  [hh1_aileron_pos] -> Signal Mux/45
  [hh1_aileron_unsat] -> Signal Mux/44
  [hh1_roll_rate_feedback] -> Signal Mux/43
  [hh1_integral] -> Signal Mux/42
  [hh1_xi] -> Signal Mux/41
  [hh1_proportional] -> Signal Mux/40
  [hh1_bank_error] -> Signal Mux/39
  [hh1_phi_sensor] -> Signal Mux/38
  [hh1_phi_input] -> Signal Mux/37
  [hh1_phi_noise] -> Signal Mux/36
  [hh1_phi_delayed] -> Signal Mux/35
  [hh1_p_sensor] -> Signal Mux/34
  [hh1_p_input] -> Signal Mux/33
  [hh1_p_noise] -> Signal Mux/32
  [hh1_p_delayed] -> Signal Mux/31
  [hh1_rudder_total] -> Signal Mux/30
  [hh1_rudder_total_raw] -> Signal Mux/29
  [hh1_rudder_rate] -> Signal Mux/28
  [hh1_rudder_rate_raw] -> Signal Mux/27
  [hh1_rudder_actual] -> Signal Mux/26
  [hh1_rudder_pos] -> Signal Mux/25
  [hh1_rudder_raw] -> Signal Mux/24
  [hh1_r_washout] -> Signal Mux/23
  [hh1_r_sensor] -> Signal Mux/22
  [hh1_r_input] -> Signal Mux/21
  [hh1_r_noise] -> Signal Mux/20
  [hh1_r_delayed] -> Signal Mux/19
  [hh1_rudder_pilot] -> Signal Mux/18
  [hh1_aileron_pilot] -> Signal Mux/17
  [hh1_bank_command_filtered] -> Signal Mux/16
  [hh1_bank_command_limited] -> Signal Mux/15
  [hh1_bank_command_raw] -> Signal Mux/14
  [hh1_heading_error] -> Signal Mux/13
  [hh1_heading_difference] -> Signal Mux/12
  [hh1_heading_sensor] -> Signal Mux/11
  [hh1_heading_input] -> Signal Mux/10
  [hh1_heading_noise] -> Signal Mux/9
  [hh1_heading_bias] -> Signal Mux/8
  [hh1_psi_delayed] -> Signal Mux/7
  [hh1_heading_command] -> Signal Mux/6
  [hh1_psi] -> Signal Mux/5
  [hh1_phi] -> Signal Mux/4
  [hh1_r] -> Signal Mux/3
  [hh1_p] -> Signal Mux/2
  [hh1_beta] -> Signal Mux/1

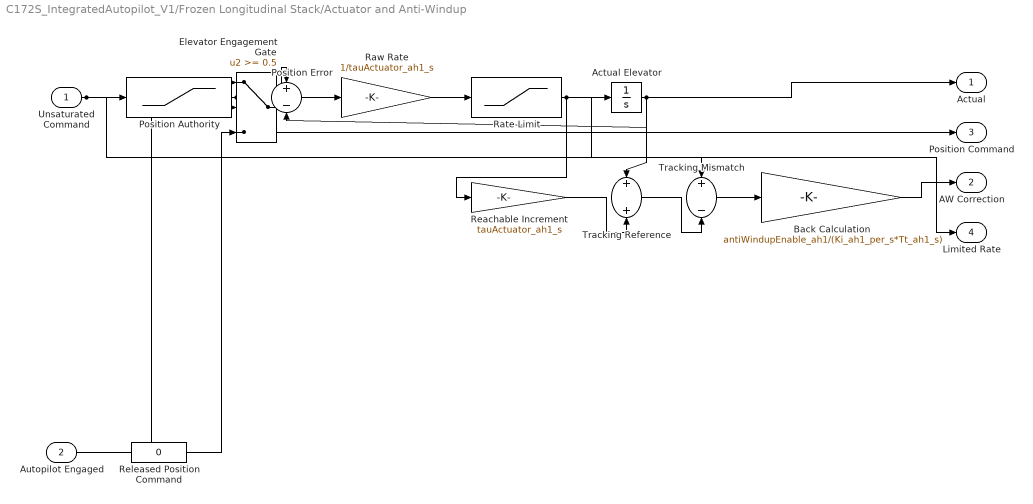
== system C172S_IntegratedAutopilot_V1/Frozen Longitudinal Stack/Actuator and Anti-Windup ==
  Unsaturated Command : Inport
  Autopilot Engaged : Inport  Port=2
  Actual Elevator : Integrator  InitialCondition=deltaE0_ah1
  Back Calculation : Gain  Gain=antiWindupEnable_ah1/(Ki_ah1_per_s*Tt_ah1_s)
  Elevator Engagement Gate : Switch  Threshold=0.5  SaturateOnIntegerOverflow=off  InputSameDT=off
  Position Authority : Saturate  UpperLimit=deltaEUpper_ah1_rad  LowerLimit=deltaELower_ah1_rad
  Position Error : Sum  Inputs=+-
  Rate Limit : Saturate  UpperLimit=deltaERate_ah1_radps  LowerLimit=-deltaERate_ah1_radps
  Raw Rate : Gain  Gain=1/tauActuator_ah1_s
  Reachable Increment : Gain  Gain=tauActuator_ah1_s
  Released Position Command : Constant  Value=0
  Tracking Mismatch : Sum  Inputs=+-
  Tracking Reference : Sum
  Actual : Outport
  AW Correction : Outport  Port=2
  Position Command : Outport  Port=3
  Limited Rate : Outport  Port=4
  wires:
  Back Calculation/1 -> AW Correction/1
  Tracking Mismatch/1 -> Back Calculation/1
  Tracking Reference/1 -> Tracking Mismatch/2
  Reachable Increment/1 -> Tracking Reference/2
  Actual Elevator/1 -> Actual/1, Tracking Reference/1, Position Error/2
  Rate Limit/1 -> Limited Rate/1, Reachable Increment/1, Actual Elevator/1
  Raw Rate/1 -> Rate Limit/1
  Position Error/1 -> Raw Rate/1
  Position Authority/1 -> Position Command/1, Elevator Engagement Gate/1
  Unsaturated Command/1 -> Tracking Mismatch/1, Position Authority/1
  Autopilot Engaged/1 -> Elevator Engagement Gate/2
  Released Position Command/1 -> Elevator Engagement Gate/3
  Elevator Engagement Gate/1 -> Position Error/1

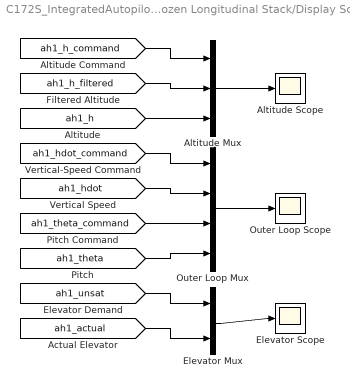
== system C172S_IntegratedAutopilot_V1/Frozen Longitudinal Stack/Display Scopes ==
  Altitude Mux : Mux  Inputs=3
  Altitude Scope : Scope
  Elevator Mux : Mux  Inputs=2
  Elevator Scope : Scope
  Outer Loop Mux : Mux
  Outer Loop Scope : Scope
  wires:
  Elevator Mux/1 -> Elevator Scope/1
  [ah1_actual] -> Elevator Mux/2
  [ah1_unsat] -> Elevator Mux/1
  Outer Loop Mux/1 -> Outer Loop Scope/1
  [ah1_theta] -> Outer Loop Mux/4
  [ah1_theta_command] -> Outer Loop Mux/3
  [ah1_hdot] -> Outer Loop Mux/2
  [ah1_hdot_command] -> Outer Loop Mux/1
  Altitude Mux/1 -> Altitude Scope/1
  [ah1_h] -> Altitude Mux/3
  [ah1_h_filtered] -> Altitude Mux/2
  [ah1_h_command] -> Altitude Mux/1

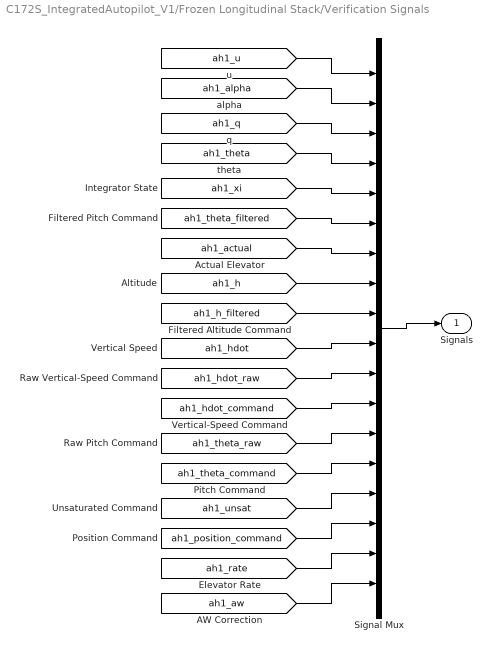
== system C172S_IntegratedAutopilot_V1/Frozen Longitudinal Stack/Verification Signals ==
  Signal Mux : Mux  Inputs=18
  Signals : Outport
  wires:
  Signal Mux/1 -> Signals/1
  [ah1_aw] -> Signal Mux/18
  [ah1_rate] -> Signal Mux/17
  [ah1_position_command] -> Signal Mux/16
  [ah1_unsat] -> Signal Mux/15
  [ah1_theta_command] -> Signal Mux/14
  [ah1_theta_raw] -> Signal Mux/13
  [ah1_hdot_command] -> Signal Mux/12
  [ah1_hdot_raw] -> Signal Mux/11
  [ah1_hdot] -> Signal Mux/10
  [ah1_h_filtered] -> Signal Mux/9
  [ah1_h] -> Signal Mux/8
  [ah1_actual] -> Signal Mux/7
  [ah1_theta_filtered] -> Signal Mux/6
  [ah1_xi] -> Signal Mux/5
  [ah1_theta] -> Signal Mux/4
  [ah1_q] -> Signal Mux/3
  [ah1_alpha] -> Signal Mux/2
  [ah1_u] -> Signal Mux/1
